simulink model "Model_hibrido_Serial_Simul"  (R2013a)
settings: Solver=ode45  StartTime=0.0  StopTime=3000  FixedStep=.05  MaxStep=0.05  RelTol=1e-3
libraries: aerolibutil x2, vrlib x2, aerolibtransform2 x1, instrumentlib x1
settings Model: Creator=Daniel  LastModifiedBy=Daniel

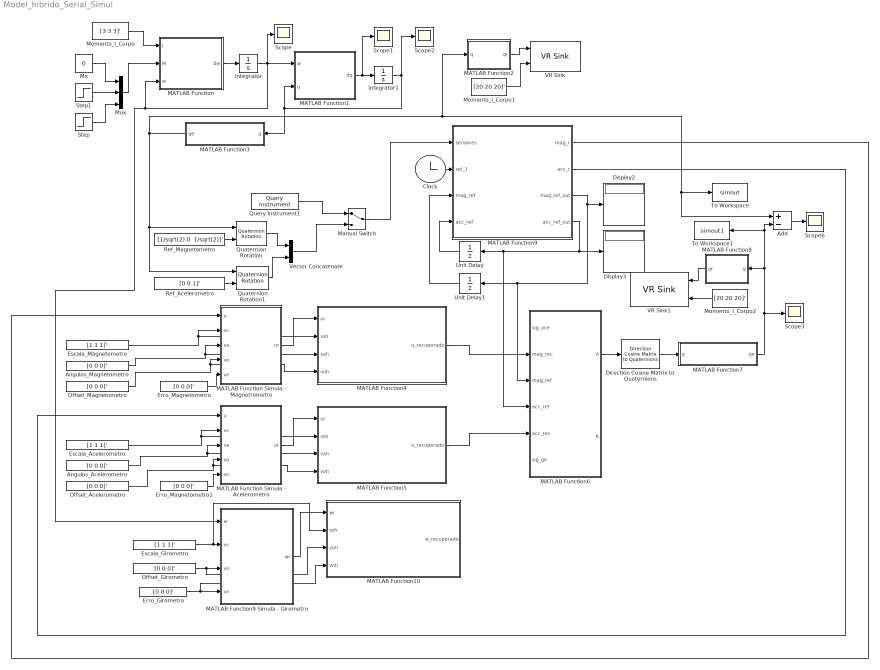
== system Model_hibrido_Serial_Simul ==
  Add : Sum  Inputs=+-
  Angulos_Acelerometro : Constant  Value=[0 0 0]'
  Angulos_Magnetometro : Constant  Value=[0 0 0]'
  Clock : Clock
  Direction Cosine Matrix to Quaternions : aerolibtransform2/Direction Cosine Matrix  to Quaternions
  Display2 : Display
  Display3 : Display
  Erro_Girometro : Constant  Value=[0 0 0]'
  Erro_Magnetometro : Constant  Value=[0 0 0]'
  Erro_Magnetometro1 : Constant  Value=[0 0 0]'
  Escala_Acelerometro : Constant  Value=[1 1 1]'
  Escala_Girometro : Constant  Value=[1 1 1]'
  Escala_Magnetometro : Constant  Value=[1 1 1]'
  Integrator : Integrator  InitialCondition=[0 0 0]
  Integrator1 : Integrator  InitialCondition=[1 0 0 0]
  MATLAB Function : MATLAB Function  TreatAsAtomicUnit=on
  MATLAB Function Simula - Acelerometro : MATLAB Function  TreatAsAtomicUnit=on
  MATLAB Function Simula - Magnetrometro : MATLAB Function  TreatAsAtomicUnit=on
  MATLAB Function1 : MATLAB Function  TreatAsAtomicUnit=on
  MATLAB Function10 : MATLAB Function  TreatAsAtomicUnit=on
  MATLAB Function2 : MATLAB Function  TreatAsAtomicUnit=on
  MATLAB Function3 : MATLAB Function  TreatAsAtomicUnit=on
  MATLAB Function4 : MATLAB Function  TreatAsAtomicUnit=on
  MATLAB Function5 : MATLAB Function  TreatAsAtomicUnit=on
  MATLAB Function6 : MATLAB Function  TreatAsAtomicUnit=on
  MATLAB Function7 : MATLAB Function  TreatAsAtomicUnit=on
  MATLAB Function8 : MATLAB Function  TreatAsAtomicUnit=on
  MATLAB Function9 : MATLAB Function  TreatAsAtomicUnit=on
  MATLAB Function9 Simula - Girometro : MATLAB Function  TreatAsAtomicUnit=on
  Manual Switch : ManualSwitch
  Momento_I_Corpo : Constant  Value=[3 3 3]'
  Momento_I_Corpo1 : Constant  Value=[20 20 20]'
  Momento_I_Corpo2 : Constant  Value=[20 20 20]'
  Mux : Mux  Inputs=3
  Mx : Constant  Value=0
  Offset_Acelerometro : Constant  Value=[0 0 0]'
  Offset_Girometro : Constant  Value=[0 0 0]'
  Offset_Magnetometro : Constant  Value=[0 0 0]'
  Quaternion Rotation : aerolibutil/Quaternion Rotation
  Quaternion Rotation1 : aerolibutil/Quaternion Rotation
  Query Instrument1 : instrumentlib/Query Instrument  sampleTime=0.05  isWorkspaceObject=off  timeout=2  inputBufferSize=512  protocol=Serial  serialPort=COM4  baudRate=115200  gpibVendor=Advantech  boardIndex=0  primaryAddress=1  secondaryAddress=0  visaVendor=Agilent  visaSerialPort=0  chassisIndex=0  logicalAddress=0  tcpRemoteHost='127.0.0.1'  tcpRemotePort=4500  udpRemoteHost='127.0.0.1'  udpRemotePort=9090  visaTCPBoardIndex=0  visaTCPRemoteHost='127.0.0.1'  usbBoardIndex=0  usbManufID=0  usbModelCode=0  usbSerialNumber=0  initAction=None  initCommand='DATA:SOURCE CH1'  initFunction=get  queryCommand='@'  responseFormat=ASCII  asciiFormatting='%d %d %d %d %d %d'  precision=16-bit integer  byteOrder=Little endian  valuesToRead=18  removeBytes=off  afterOutputAction=Repeat query for new data  enableFrames=on  frameSize=6
  Ref_Acelerometro : Constant  Value=[0 0 1]'
  Ref_Magnetometro : Constant  Value="[1/sqrt(2) 0  1/sqrt(2)]'"
  Scope{,1..3,6} (5 alike) : Scope
      Scope2 settings: SaveName=ScopeData2
      Scope3 settings: YMin=-1  YMax=1  SaveName=ScopeData3
      Scope6 settings: YMin=-4e-11  YMax=4e-11  SaveName=ScopeData6  MaxDataPoints=50000
  Step : Step  Before=1  After=0  SampleTime=0
  Step1 : Step  Before=.2  After=0  SampleTime=0
  To Workspace : ToWorkspace  VariableName=simout  SampleTime=-1
  To Workspace1 : ToWorkspace  VariableName=simout1  SampleTime=-1
  Unit Delay : UnitDelay  InitialCondition=[0 0 0]'  SampleTime=-1
  Unit Delay1 : UnitDelay  InitialCondition=[0 0 0]'  SampleTime=-1
  VR Sink : vrlib/VR Sink  InstantiateOnLoad=on  SampleTime=-1  ViewEnable=on  RemoteChange=off  RemoteView=off  FieldsWritten=H.rotation.4.1.1.double#H.scale.3.1.1.double  WorldFileName=C:\Users\Daniel\Desktop\TCC Daniel\Arquivos WRL\teste_combinado.wrl  AutoView=off  VideoDimensions=[]  AllowVariableSize=off
  VR Sink1 : vrlib/VR Sink  InstantiateOnLoad=on  SampleTime=-1  ViewEnable=on  RemoteChange=off  RemoteView=off  FieldsWritten=H.rotation.4.1.1.double#H.scale.3.1.1.double  WorldFileName=C:\Users\Daniel\Desktop\TCC Daniel\Arquivos WRL\teste_combinado2.wrl  AutoView=off  VideoDimensions=[]  AllowVariableSize=off
  Vector Concatenate : Concatenate
  wires:
  Momento_I_Corpo/1 -> MATLAB Function/1(I)
  Mux/1 -> MATLAB Function/2(M)
  MATLAB Function/1(dw) -> Integrator/1
  Integrator/1 -> MATLAB Function1/1(w), Scope/1, MATLAB Function9 Simula - Girometro/1(w), MATLAB Function/3(w)
  MATLAB Function1/1(dq) -> Integrator1/1, Scope1/1
  Integrator1/1 -> MATLAB Function3/1(q), MATLAB Function1/2(q), Scope2/1
  MATLAB Function3/1(qe) -> Quaternion Rotation/1, Quaternion Rotation1/1, MATLAB Function2/1(q), Add/1, To Workspace/1
  Ref_Acelerometro/1 -> Quaternion Rotation1/2
  Erro_Magnetometro/1 -> MATLAB Function Simula - Magnetrometro/5(vn)
  Erro_Magnetometro1/1 -> MATLAB Function Simula - Acelerometro/5(vn)
  Offset_Magnetometro/1 -> MATLAB Function Simula - Magnetrometro/4(vo), MATLAB Function4/4(voh)
  Escala_Acelerometro/1 -> MATLAB Function Simula - Acelerometro/2(vs), MATLAB Function5/2(vsh)
  Angulos_Acelerometro/1 -> MATLAB Function Simula - Acelerometro/3(va), MATLAB Function5/3(vah)
  Offset_Acelerometro/1 -> MATLAB Function Simula - Acelerometro/4(vo), MATLAB Function5/4(voh)
  MATLAB Function Simula - Magnetrometro/1(ur) -> MATLAB Function4/1(ur)
  MATLAB Function Simula - Acelerometro/1(ur) -> MATLAB Function5/1(ur)
  Escala_Magnetometro/1 -> MATLAB Function Simula - Magnetrometro/2(vs), MATLAB Function4/2(vsh)
  Angulos_Magnetometro/1 -> MATLAB Function Simula - Magnetrometro/3(va), MATLAB Function4/3(vah)
  MATLAB Function5/1(u_recuperado) -> MATLAB Function6/5(acc_rec)
  MATLAB Function4/1(u_recuperado) -> MATLAB Function6/2(mag_rec)
  MATLAB Function6/1(A) -> Direction Cosine Matrix to Quaternions/1
  MATLAB Function7/1(qe) -> Add/2, To Workspace1/1, MATLAB Function8/1(q), Scope3/1
  MATLAB Function9 Simula - Girometro/1(wr) -> MATLAB Function10/1(wr)
  Escala_Girometro/1 -> MATLAB Function10/2(vsh), MATLAB Function9 Simula - Girometro/2(vs)
  Offset_Girometro/1 -> MATLAB Function10/3(voh), MATLAB Function9 Simula - Girometro/3(vo)
  Direction Cosine Matrix to Quaternions/1 -> MATLAB Function7/1(q)
  Erro_Girometro/1 -> MATLAB Function10/4(vnh), MATLAB Function9 Simula - Girometro/4(vn)
  Unit Delay/1 -> MATLAB Function9/4(acc_ref)
  Unit Delay1/1 -> MATLAB Function9/3(mag_ref)
  Quaternion Rotation/1 -> Vector Concatenate/1
  Quaternion Rotation1/1 -> Vector Concatenate/2
  MATLAB Function9/3(mag_ref_out) -> Display2/1, MATLAB Function6/3(mag_ref), Unit Delay1/1
  MATLAB Function9/4(acc_ref_out) -> Unit Delay/1, MATLAB Function6/4(acc_ref), Display3/1
  Add/1 -> Scope6/1
  Clock/1 -> MATLAB Function9/2(sel_1)
  Momento_I_Corpo1/1 -> VR Sink/2
  MATLAB Function2/1(qr) -> VR Sink/1
  MATLAB Function9/1(mag_r) -> MATLAB Function Simula - Magnetrometro/1(u)
  MATLAB Function9/2(acc_r) -> MATLAB Function Simula - Acelerometro/1(u)
  Step/1 -> Mux/3
  Step1/1 -> Mux/2
  Mx/1 -> Mux/1
  Ref_Magnetometro/1 -> Quaternion Rotation/2
  MATLAB Function8/1(qr) -> VR Sink1/1
  Momento_I_Corpo2/1 -> VR Sink1/2
  Vector Concatenate/1 -> Manual Switch/2
  Query Instrument1/1 -> Manual Switch/1
  Manual Switch/1 -> MATLAB Function9/1(sensores)

== matlab function Model_hibrido_Serial_Simul/MATLAB Function1 ==
  data: w input; dq output; q input
function dq = cinematica(w,q)
%#eml
wx = w(1);
wy = w(2);
wz = w(3);

q = q/norm(q);

qteta = q(1);
qx = q(2);
qy = q(3);
qz = q(4);

W = [0 -wx -wy -wz; wx 0 wz -wy; wy -wz 0 wx; wz wy -wx 0];
%W=[0 wz -wy wx; -wz 0 wx wy; wy -wx 0 wz; -wx -wy -wz 0];
dq=0.5*W*[qteta qx qy qz]';

== matlab function Model_hibrido_Serial_Simul/MATLAB Function ==
  data: I input; dw output; M input; w input
function dw  = Eq_Euler(I,M,w)
%#eml
wx = w(1);
wy = w(2);
wz = w(3);

Ix = I(1);
Iy = I(2);
Iz = I(3);

Mx = M(1);
My = M(2);
Mz = M(3);

dwx = (Mx - wy*wz*(Iz - Iy))/Ix;
dwy = (My - wx*wz*(Ix - Iz))/Iy;
dwz = (Mz - wx*wy*(Iy - Ix))/Iz;

dw=[dwx dwy dwz]';

== matlab function Model_hibrido_Serial_Simul/MATLAB Function2 ==
  data: q input; qr output
function qr = ajusta_q(q)
%#eml

q = q/(norm(q));
v = [q(2) q(3) q(4)] / norm([q(2) q(3) q(4)]);
ang = acos(q(1))*2;

qr = [v ang];

== matlab function Model_hibrido_Serial_Simul/MATLAB Function3 ==
  data: q input; qe output
function qe = tira_redundancia(q)
qe = zeros(4,1);
%#eml

if q(1)<0
    qe = -q;
else
    qe = q;
end

== matlab function Model_hibrido_Serial_Simul/MATLAB Function Simula - Magnetrometro ==
  data: u input; ur output; vs input; va input; vo input; vn input
function ur = triad_model(u,vs,va,vo,vn)
%#eml

rho = va(1);
phi = va(2);
lambda = va(3);

S = diag(vs);
T = [1 0 0; sin(rho) cos(rho) 0;...
    sin(phi)*cos(lambda) sin(lambda)*cos(phi) cos(phi)*cos(lambda)];

ur = S*T*u + vo + vn;

== matlab function Model_hibrido_Serial_Simul/MATLAB Function Simula - Acelerometro ==
  data: u input; ur output; vs input; va input; vo input; vn input
function ur = triad_model(u,vs,va,vo,vn)
%#eml

rho = va(1);
phi = va(2);
lambda = va(3);

S = diag(vs);
T = [1 0 0; sin(rho) cos(rho) 0;...
    sin(phi)*cos(lambda) sin(lambda)*cos(phi) cos(phi)*cos(lambda)];

ur = S*T*u + vo + vn;

== matlab function Model_hibrido_Serial_Simul/MATLAB Function4 ==
  data: ur input; u_recuperado output; vsh input; vah input; voh input
function u_recuperado = inv_triad_model(ur,vsh,vah,voh)
%#eml

rho = vah(1);
phi = vah(2);
lambda = vah(3);

T_inv = [1 0 0; -tan(rho) 1/cos(rho) 0;...
    tan(rho)*tan(lambda)-tan(phi) -tan(lambda)/cos(rho) 1/(cos(lambda)*cos(phi))];
S_inv = inv(diag(vsh));

u_recuperado = T_inv*S_inv*(ur - voh);

== matlab function Model_hibrido_Serial_Simul/MATLAB Function5 ==
  data: ur input; u_recuperado output; vsh input; vah input; voh input
function u_recuperado = inv_triad_model(ur,vsh,vah,voh)
%#eml

rho = vah(1);
phi = vah(2);
lambda = vah(3);

T_inv = [1 0 0; -tan(rho) 1/cos(rho) 0;...
    tan(rho)*tan(lambda)-tan(phi) -tan(lambda)/cos(rho) 1/(cos(lambda)*cos(phi))];
S_inv = inv(diag(vsh));

u_recuperado = T_inv*S_inv*(ur - voh);

== matlab function Model_hibrido_Serial_Simul/MATLAB Function6 ==
  data: sig_ace input; A output; mag_rec input; mag_ref input; acc_ref input; acc_rec input; sig_gir input; R output
function [A,R] = TRIAD(sig_ace,mag_rec,mag_ref,acc_ref,acc_rec,sig_gir)

% ========== Função de Determinação de Atitude ===========
% ========== Algoritmo TRIAD ===========
% Os parâmetros de Entrada são:
% V1 : vetor de referência V1
V1 = acc_ref;
% V2 : vetor de referência V2
V2 = mag_ref;
% W1 : vetor de observação W1
W1 = acc_rec;
% W2 : vetor de observação W2
W2 = mag_rec;
% SigTo1 : desvio padrão das observação do Acelerômetro
SigTot1 = sig_ace;
% SigTo2 : desvio padrão das observação do Magnetômetro
SigTot2 = sig_gir;

% ========================================================
% Os parâmetros de Retorno são:
% A : matriz de atitude
% P : Covariância da atitude
% ========================================================
% --- Obtendo a Tríade de Referência
r1 = V1/norm(V1);
r2 = cross(V1,V2); % função do produto vetorial
r2 = r2 / norm(r2);
r3 = cross(r1,r2);
% --- Montando a Matriz de Referência
Mref = [r1 r2 r3];

% --- Obtendo a tríade de observação
s1 = W1/norm(W1);
s2 = cross(W1,W2);
s2 = s2 / norm(s2);
s3 = cross(s1,s2);
% --- Montando a Matriz de Observação
Mobs = [s1 s2 s3];
% --- Atitude pelo TRIAD
A = Mobs * Mref';
%--------------------------------------------------------------------------
% Obtendo a covariância da atitude (P = P + AP AT)
R = SigTot1^2 * eye(3) + ...
    (1/norm(cross(W1,W2)))^2 * (SigTot1^2* (W1'*W2) * (W1*W2' + W2*W1')...
    + (SigTot2^2 - SigTot1^2)*W1*W1');

%--------------------------------------------------------------------------

== matlab function Model_hibrido_Serial_Simul/MATLAB Function7 ==
  data: q input; qe output
function qe = tira_redundancia(q)
qe = zeros(4,1);
%#eml

if q(1)<0
    qe = -q;
else
    qe = q;
end

== matlab function Model_hibrido_Serial_Simul/MATLAB Function8 ==
  data: q input; qr output
function qr = ajusta_q(q)
%#eml

q = q/(norm(q));
v = [q(2) q(3) q(4)] / norm([q(2) q(3) q(4)]);
ang = acos(q(1))*2;

qr = [v ang];

== matlab function Model_hibrido_Serial_Simul/MATLAB Function9 Simula - Girometro ==
  data: w input; wr output; vs input; vo input; vn input
function wr = gyro_model(w,vs,vo,vn)
%#eml

S = diag(vs);

wr = S*w + vo + vn*randn;

== matlab function Model_hibrido_Serial_Simul/MATLAB Function10 ==
  data: wr input; w_recuperado output; vsh input; voh input; vnh input
function w_recuperado = inv_gyro_model(wr,vsh,voh,vnh)
%#eml

S_inv = inv(diag(vsh));

w_recuperado = S_inv*(wr - voh);

== matlab function Model_hibrido_Serial_Simul/MATLAB Function9 ==
  data: sensores input; sel_1 input; mag_r output; acc_r output; mag_ref input; acc_ref input; mag_ref_out output; acc_ref_out output
function [mag_r, acc_r, mag_ref_out, acc_ref_out] = fcn(sensores, sel_1, mag_ref, acc_ref)
%#codegen

mag_ref_out = zeros(3,1);
acc_ref_out = zeros(3,1);

mag_x = sensores(1);
mag_y = sensores(2);
mag_z = sensores(3);

acc_x = sensores(4);
acc_y = sensores(5);
acc_z = sensores(6);

mag_ref_out = mag_ref;
acc_ref_out = acc_ref;

if sel_1 == 0
mag_ref_out = [mag_x mag_y mag_z]';
acc_ref_out = [acc_x acc_y acc_z]';
end

mag_r = [mag_x mag_y mag_z]';
acc_r = [acc_x acc_y acc_z]';
